simulink model "DCDC_3_5"  (R2012b)
settings: Solver=ode23  StartTime=0.0  StopTime=1370  FixedStep=0.1  MaxStep=0.005  RelTol=1e-6
undefined symbols (not defined in the file): Ion, Lithium
libraries: powerlib x12, simulink x4, electricdrivelib x1
settings Model: Creator=Administrator  LastModifiedBy=Administrator
settings DataIOCC: SignalLoggingSaveFormat=ModelDataLogs
settings DebuggingCC: FcnCallInpInsideContextMsg=UseLocalSettings  StrictBusMsg=Warning
settings GRTTargetCC: CombineOutputUpdateFcns=off  GRTInterface=on

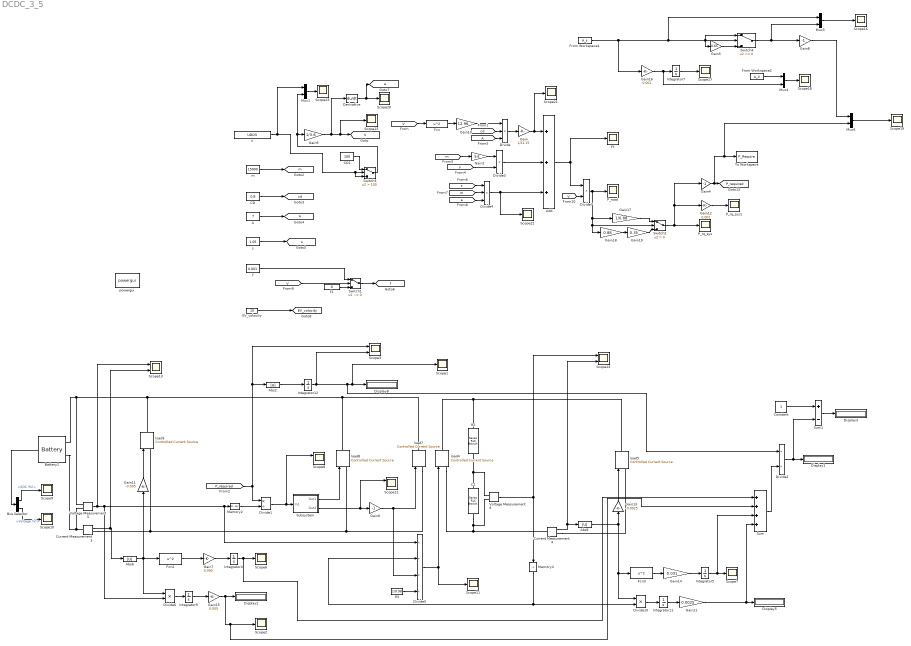
== system DCDC_3_5 ==
  A : Constant  Value=7
  Abs2 : Abs
  Abs6 : Abs
  Abs9 : Abs
  Add : Sum  Inputs=+++
  Battery2 : electricdrivelib/Extra Sources/Battery  BatType=Lithium-Ion  ShowDetailedParameters=on  NomV=576  NomQ=160  SOC=90  PresetModel=off  MaxQ=160  FullV=670.4566  Dis_rate=69.5652  R=0.09  Normal_OP=144.6957  expZone="[622.3023       7.86087]"  Dis_Char=off  current=[1.5 3]  Units=Ampere-hour  Batt_Tr=30
  Bus Selector : BusSelector  OutputSignals=SOC (%),Voltage (V)
  C2 : powerlib/Elements/Series RLC Branch  LConnTagsString=__new0  RConnTagsString=__new0  BranchType=C  Resistance=1  Inductance=1e-3  SetiL0=off  InitialCurrent=0  Capacitance=28.3  Setx0=on  InitialVoltage=400  Measurements=Branch voltage
  CD : Constant  Value=0.8
  CD1 : Constant  Value=100
  Constant : Constant
  Current Measurement3 : powerlib/Measurements/Current Measurement  PhasorSimulation=off  OutputType=Complex  PSBequivalent=0
  Current Measurement4 : powerlib/Measurements/Current Measurement  PhasorSimulation=off  OutputType=Complex  PSBequivalent=0
  Derivative : Derivative
  Display{1..3,5,8} (5 alike) : Display
  Divide : Product  Inputs=***
  Divide1 : Product  Inputs=*/
  Divide{3,6..7,10} (4 alike) : Product  Inputs=**
  Divide2 : Product  Inputs=/*
  Divide4 : Product  Inputs=***
  Divide5 : Product  Inputs=*/**
  E3 : Constant  Value=1/0.98
  EV_volocity : Constant  Value=10
  Fcn : Fcn  Expr=u^2
  Fcn2 : Fcn  Expr=u^2
  Fcn3 : Fcn  Expr=u^2
  From Workspace2 : FromWorkspace  VariableName=A_V  SampleTime=0
  From Workspace4 : FromWorkspace  VariableName=A_t  SampleTime=0
  Ft : Scope
      settings: SaveName=ScopeData14
  Gain : Gain  Gain=1/21.15
  Gain10 : Gain  Gain=12.96
  Gain11 : Gain  Gain=-0.005
  Gain12 : Gain  Gain=0.001
  Gain13 : Gain  Gain=-0.0025
  Gain14 : Gain  Gain=0.031
  Gain15 : Gain  Gain=0.005
  Gain16 : Gain  Gain=0.001
  Gain17 : Gain  Gain=1/0.88
  Gain18 : Gain  Gain=0.88
  Gain19 : Gain  Gain=0.35
  Gain2 : Gain  Gain=9.8
  Gain21 : Gain  Gain=0.0025
  Gain4 : Gain  Gain=-1
  Gain5 : Gain  Gain=0.65
  Gain6 : Gain  Gain=-1
  Gain7 : Gain  Gain=0.090
  Gain8 : Gain  Gain=-1
  Gain9 : Gain  Gain=1/3.6
  Integrator{4..5,7,9,11..12} (6 alike) : Integrator
  Memory2 : Memory  X0=380
  Memory4 : Memory  X0=380
  Mux{1,4..6} (4 alike) : Mux  Inputs=2
  P_road : Scope
      settings: SaveName=P_road
  P_rq_sys : Scope
      settings: SaveName=ScopeData15
  P_rq_sys1 : Scope
      settings: SaveName=ScopeData16
  R2 : powerlib/Elements/Series RLC Branch  LConnTagsString=__new0  RConnTagsString=__new0  BranchType=R  Resistance=0.031  Inductance=1e-3  SetiL0=off  InitialCurrent=0  Capacitance=1e-6  Setx0=off  InitialVoltage=0  Measurements=None
  Scope{1..2,6..7,9..11,15..23} (16 alike) : Scope
      Scope10 settings: SaveName=ScopeData11
      Scope11 settings: SaveName=ScopeData4
      Scope15 settings: SaveName=ScopeData17
      Scope16 settings: SaveName=ScopeData18
      Scope17 settings: SaveName=ScopeData19
      Scope18 settings: SaveName=ScopeData20
      Scope19 settings: SaveName=ScopeData21
      Scope20 settings: SaveName=ScopeData22
      Scope21 settings: SaveName=ScopeData23
      Scope22 settings: SaveName=ScopeData24
      Scope23 settings: SaveName=ScopeData25
      Scope6 settings: SaveName=ScopeData9
      Scope7 settings: SaveName=ScopeData10
      Scope9 settings: SaveName=ScopeData8
  Scope{3,8,12..14} (5 alike) : Scope  NumInputPorts=2
      Scope12 settings: YMin=-5~-5  YMax=5~5  SaveName=ScopeData5
      Scope13 settings: YMin=-5~-5  YMax=5~5  SaveName=ScopeData12
      Scope14 settings: YMin=-5~-5  YMax=5~5  SaveName=ScopeData13
      Scope3 settings: YMin=-5~-5  YMax=5~5  SaveName=ScopeData2
      Scope8 settings: YMin=-5~-5  YMax=5~5  SaveName=ScopeData3
  Subsystem : Subsystem
  Sum : Sum  Inputs=++++
  Sum1 : Sum  Inputs=+-
  Switch1 : Switch  Criteria=u2 ~= 0
  Switch2 : Switch  Criteria=u2 > Threshold
  Switch3 : Switch  Criteria=u2 > Threshold  Threshold=100
  Switch4 : Switch
  To Workspace : ToWorkspace  VariableName=P_Require  SampleTime=-1
  V : FromWorkspace  VariableName=UDDS  SampleTime=0
  Voltage Measurement5 : powerlib/Measurements/Voltage Measurement  PhasorSimulation=off  OutputType=Complex  PSBequivalent=0
  Voltage Measurement6 : powerlib/Measurements/Voltage Measurement  PhasorSimulation=off  OutputType=Complex  PSBequivalent=0
  f : Constant  Value=0.001
  f1 : Constant  Value=0
  load{3..5,7..8} (5 alike) : powerlib/Electrical Sources/Controlled Current Source  Initialize=on  Source_Type=AC  Amplitude=0  Phase=0  Frequency=0  Measurements=None
  m : Constant  Value=15000
  powergui : powerlib/powergui  Priority=1  SimulationMode=Discrete  SolverType=Tustin  SampleTime=0.01  frequency=60  SPID=off  DisableSnubberDevices=off  DisableRonSwitches=off  DisableVfSwitches=off  SwTol=0  Interpol=off  DisplayEquations=off  FunctionMessages=off  frequencyindice=0  Pbase=100e6  ErrMax=1e-4  Iterations=50  UnitsV=kV  UnitsW=MW  echomessages=off  HookPort=off  EnableUseOfTLC=off  x0status=blocks  RestoreLinks=warning  ResistiveCurrentMeasurement=off  Ylog=off  Xlog=on  ShowGrid=off  save=off  variable=ZData  ZoomFFT=off  StartTime=0.0  cycles=1  DisplayStyle=1  FreqAxis=off  MaxFrequency=1000  frequencyindicesteady=1  display=off  methode=off
  s : Constant  Value=1.05
  tag scope: A=global, EV_volocity=global, P_required=global, V=global, a=global, cd=global, f=global, m=global, s=global
  wires:
  [P_required] -> Divide1/1, Abs2/1, Scope3/1
  Voltage Measurement5/1 -> Scope13/1, Divide6/2, Divide5/1, Memory2/1
  Divide1/1 -> Scope8/1, Subsystem/1(In1)
  Subsystem/1(Out1) -> load8/1
  Current Measurement3/1 -> Scope13/2, Abs6/1
  Abs6/1 -> Divide6/1, Fcn2/1, Gain11/1
  Fcn2/1 -> Gain7/1
  Gain7/1 -> Integrator4/1
  Integrator4/1 -> Sum/1, Scope6/1
  Gain13/1 -> load5/1
  Gain11/1 -> load3/1
  Fcn3/1 -> Gain14/1
  Gain14/1 -> Integrator5/1
  Integrator5/1 -> Sum/3, Scope7/1
  Current Measurement4/1 -> Abs9/1, Scope14/2
  Abs9/1 -> Divide10/1, Fcn3/1, Gain13/1
  Voltage Measurement6/1 -> Scope14/1, Memory4/1
  E3/1 -> Divide5/4
  Divide5/1 -> load4/1, Scope11/1
  Subsystem/2(Out2) -> Scope12/1, Gain6/1
  Gain6/1 -> Divide5/3, load7/1
  Divide6/1 -> Integrator9/1
  Integrator9/1 -> Gain15/1
  Gain15/1 -> Sum/2, Scope2/1, Display2/1
  Divide10/1 -> Integrator11/1
  Integrator11/1 -> Gain21/1
  Gain21/1 -> Sum/4, Display5/1
  Memory2/1 -> Divide1/2
  Memory4/1 -> Divide10/2, Divide5/2
  Integrator12/1 -> Scope3/2, Divide2/1, Scope1/1, Display8/1
  Abs2/1 -> Integrator12/1
  Battery2/1 -> Bus Selector/1
  Bus Selector/1 -> Scope9/1  "<SOC (%)>"
  Bus Selector/2 -> Scope10/1  "<Voltage (V)>"
  Sum/1 -> Divide2/2
  Divide2/1 -> Sum1/2, Display1/1
  Constant/1 -> Sum1/1
  Sum1/1 -> Display3/1
  V/1 -> Mux1/1, Switch3/3, Switch3/2
  m/1 -> [m]
  CD/1 -> [cd]
  A/1 -> [A]
  s/1 -> [s]
  Derivative/1 -> Scope20/1, [a]
  [V] -> Fcn/1
  Fcn/1 -> Gain10/1
  [cd] -> Divide/2
  Divide/1 -> Gain/1
  Gain/1 -> Add/1, Scope21/1
  [m] -> Gain2/1
  Gain2/1 -> Divide3/1
  [f] -> Divide3/2
  [A] -> Divide/3
  Divide3/1 -> Add/2
  [s] -> Divide4/1
  [m] -> Divide4/2
  [a] -> Divide4/3
  Divide4/1 -> Add/3, Scope22/1
  Add/1 -> Ft/1, Divide7/1
  f/1 -> Switch1/1
  [V] -> Switch1/2
  f1/1 -> Switch1/3
  Switch1/1 -> [f]
  Gain9/1 -> Derivative/1, [V], Scope15/1
  [V] -> Divide7/2
  Gain10/1 -> Divide/1
  Divide7/1 -> P_road/1, Gain17/1, Switch2/2, Gain18/1
  Gain17/1 -> Switch2/1
  Gain18/1 -> Gain19/1
  Switch2/1 -> P_rq_sys/1, Gain12/1, Gain4/1
  Gain19/1 -> Switch2/3
  EV_volocity/1 -> [EV_volocity]
  Gain4/1 -> Mux6/2, To Workspace/1, [P_required]
  Gain12/1 -> P_rq_sys1/1
  CD1/1 -> Switch3/1
  Switch3/1 -> Mux1/2, Gain9/1
  Mux1/1 -> Scope23/1
  Gain16/1 -> Integrator7/1, Mux4/2
  Integrator7/1 -> Scope17/1
  From Workspace4/1 -> Gain5/1, Switch4/1, Switch4/2, Mux5/1, Gain16/1
  From Workspace2/1 -> Mux4/1
  Mux4/1 -> Scope18/1
  Switch4/1 -> Gain8/1, Mux5/2
  Gain5/1 -> Switch4/3
  Mux5/1 -> Scope16/1
  Gain8/1 -> Mux6/1
  Mux6/1 -> Scope19/1
  connections:
  R2/RConn1 -- Voltage Measurement6/LConn1 -- C2/LConn1
  load3/RConn1 -- Voltage Measurement5/LConn1 -- Battery2/LConn1 -- load7/RConn1 -- load8/RConn1
  Battery2/LConn2 -- Voltage Measurement5/LConn2 -- Current Measurement3/LConn1
  Current Measurement3/RConn1 -- load7/LConn1 -- load8/LConn1 -- load3/LConn1
  R2/LConn1 -- load5/RConn1 -- load4/RConn1
  C2/RConn1 -- Voltage Measurement6/LConn2 -- Current Measurement4/LConn1 -- load4/LConn1
  Current Measurement4/RConn1 -- load5/LConn1

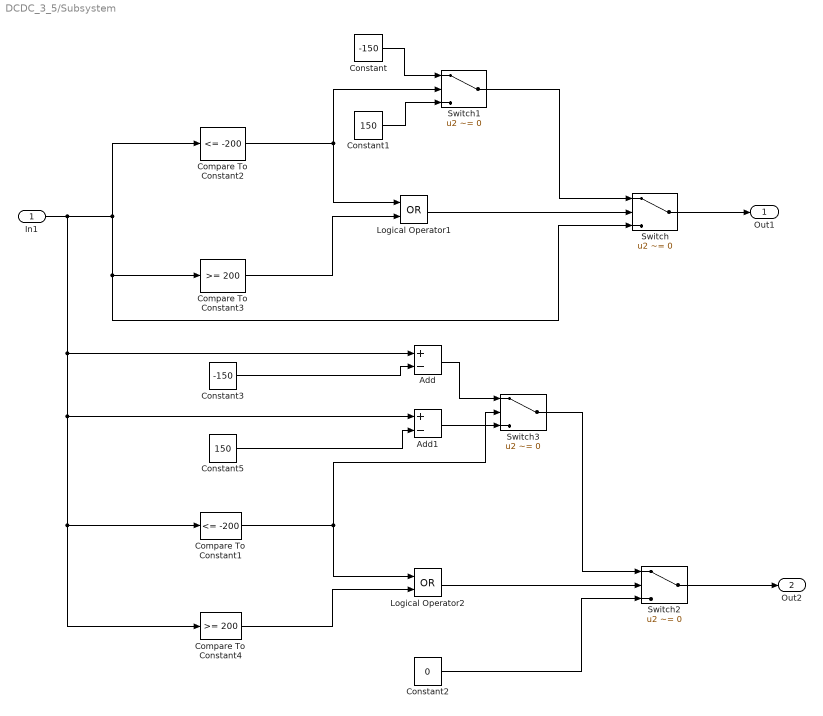
== system DCDC_3_5/Subsystem ==
  In1 : Inport
  Add : Sum  Inputs=+-
  Add1 : Sum  Inputs=+-
  Compare To Constant1 : simulink/Logic and Bit Operations/Compare To Constant  relop=<=  const=-200  OutDataTypeStr=boolean
  Compare To Constant2 : simulink/Logic and Bit Operations/Compare To Constant  relop=<=  const=-200  OutDataTypeStr=boolean  ZeroCross=off
  Compare To Constant3 : simulink/Logic and Bit Operations/Compare To Constant  relop=>=  const=200  OutDataTypeStr=boolean
  Compare To Constant4 : simulink/Logic and Bit Operations/Compare To Constant  relop=>=  const=200  OutDataTypeStr=boolean
  Constant : Constant  Value=-150
  Constant1 : Constant  Value=150
  Constant2 : Constant  Value=0
  Constant3 : Constant  Value=-150
  Constant5 : Constant  Value=150
  Logical Operator1 : Logic  Operator=OR  AllPortsSameDT=off  OutDataTypeStr=boolean
  Logical Operator2 : Logic  Operator=OR  AllPortsSameDT=off  OutDataTypeStr=boolean
  Switch{,1..3} (4 alike) : Switch  Criteria=u2 ~= 0
  Out1 : Outport
  Out2 : Outport  Port=2
  wires:
  Compare To Constant2/1 -> Switch1/2, Logical Operator1/1
  Compare To Constant3/1 -> Logical Operator1/2
  Logical Operator1/1 -> Switch/2
  Constant/1 -> Switch1/1
  Constant1/1 -> Switch1/3
  Switch1/1 -> Switch/1
  In1/1 -> Compare To Constant1/1, Compare To Constant4/1, Add1/1, Add/1, Switch/3, Compare To Constant3/1, Compare To Constant2/1
  Compare To Constant1/1 -> Logical Operator2/1, Switch3/2
  Compare To Constant4/1 -> Logical Operator2/2
  Logical Operator2/1 -> Switch2/2
  Constant2/1 -> Switch2/3
  Constant3/1 -> Add/2
  Switch3/1 -> Switch2/1
  Switch2/1 -> Out2/1
  Add/1 -> Switch3/1
  Constant5/1 -> Add1/2
  Add1/1 -> Switch3/3
  Switch/1 -> Out1/1
